simulink model "Baseline_Ctrl_Updated"  (R2020a)
settings: Solver=FixedStepAuto  StartTime=0.0  StopTime=10.0  FixedStep=DT  RelTol=1e-3  EnableMultiTasking=on
values from neighbouring files (symbols this model uses):
  K_T = 0.5e-6*pi*tp.rho*tp.R^5*tp.C_p_star/(tp.lambda_star^3)    [baseline_design.m]    (also in run_Top_Model.m)
  M_1 = K_T * Omega_1^2    [baseline_design.m]
  M_rated = 1e-6 * tp.P_rated / tp.Omega_r_rated    [baseline_design.m]
  Omega_1 = tp.Omega_r_rated * 0.9    [baseline_design.m]
  Omega_2 = tp.Omega_r_rated    [baseline_design.m]
  T_s = 0.1    [run_Top_Model.m]
  tp = turbine_params_5MW()    [baseline_design.m]    (also in run_Top_Model.m)
undefined symbols (not defined in the file or in its folder): DiscIntNeverNeededParam
settings Model: Creator=lpwoolcock  LastModifiedBy=Vince

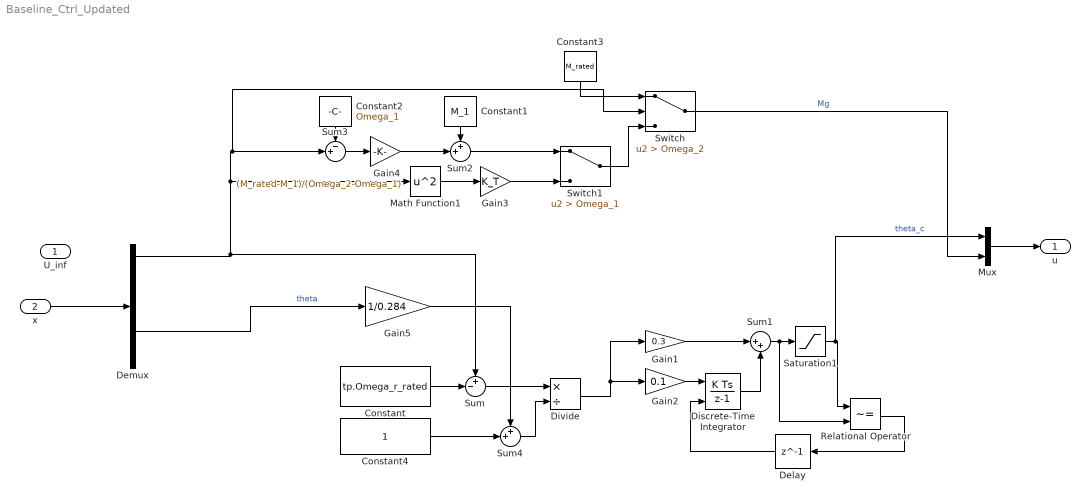
== system Baseline_Ctrl_Updated ==
  U_inf : Inport  SampleTime=T_s
  x : Inport  Port=2
  Constant : Constant  Value=tp.Omega_r_rated
  Constant1 : Constant  Value=M_1
  Constant2 : Constant  Value=Omega_1
  Constant3 : Constant  Value=M_rated
  Constant4 : Constant
  Delay : Delay  DelayLength=1
  Demux : Demux  Outputs=5
  Discrete-Time Integrator : DiscreteIntegrator  ExternalReset=level  SampleTime=T_s  ICPrevOutput=DiscIntNeverNeededParam  ICPrevScaledInput=DiscIntNeverNeededParam
  Divide : Product  Inputs=*/
  Gain1 : Gain  Gain=0.3
  Gain2 : Gain  Gain=0.1
  Gain3 : Gain  Gain=K_T
  Gain4 : Gain  Gain=(M_rated-M_1)/(Omega_2-Omega_1)
  Gain5 : Gain  Gain=1/0.284
  Math Function1 : Math  Operator=square  SaturateOnIntegerOverflow=on
  Mux : Mux  Inputs=2
  Relational Operator : RelationalOperator  Operator=~=  OutDataTypeStr=boolean  RndMeth=Simplest
  Saturation1 : Saturate  UpperLimit=inf  LowerLimit=0
  Sum : Sum  Inputs=+-|
  Sum1 : Sum  Inputs=|++
  Sum2 : Sum  Inputs=++|
  Sum3 : Sum  Inputs=-+|
  Sum4 : Sum  Inputs=++|
  Switch : Switch  Criteria=u2 > Threshold  Threshold=Omega_2
  Switch1 : Switch  Criteria=u2 > Threshold  Threshold=Omega_1
  u : Outport  SampleTime=T_s
  wires:
  Saturation1/1 -> Mux/1, Relational Operator/1  "theta_c"
  Switch/1 -> Mux/2  "Mg"
  Constant/1 -> Sum/2
  Gain2/1 -> Discrete-Time Integrator/1
  Gain1/1 -> Sum1/1
  Discrete-Time Integrator/1 -> Sum1/2
  Sum1/1 -> Relational Operator/2, Saturation1/1
  Relational Operator/1 -> Delay/1
  Delay/1 -> Discrete-Time Integrator/2
  Switch1/1 -> Switch/3
  Gain3/1 -> Switch1/3
  Math Function1/1 -> Gain3/1
  Sum2/1 -> Switch1/1
  Constant1/1 -> Sum2/1
  Gain4/1 -> Sum2/2
  Sum3/1 -> Gain4/1
  Constant2/1 -> Sum3/1
  Constant3/1 -> Switch/1
  Divide/1 -> Gain2/1, Gain1/1
  Sum/1 -> Divide/1
  Constant4/1 -> Sum4/2
  Sum4/1 -> Divide/2
  Gain5/1 -> Sum4/1
  Mux/1 -> u/1
  x/1 -> Demux/1
  Demux/4 -> Gain5/1  "theta"
  Demux/1 -> Sum/1, Math Function1/1, Switch/2, Sum3/2
